simulink model "six_plus_six_AcmsteeringV09_main_2lfrf"  (R2014a)
settings: Solver=FixedStepDiscrete  StartTime=0.0  StopTime=10.0  FixedStep=0.0005  RelTol=1e-3
InitFcn:
  | Veh_Par_wxt
undefined symbols (not defined in the file or in its folder): acc_spdctl, ag_thr, B, bra_em, bra_pre_gz2, bra_pre_gz34, bra_pre_yd, brakepre_dem_data, brakeTrq_dem_data, bratrq_max, ecucoder_acal, eff_tran, ESP_switch, G, guzhang_lf, guzhang_lm, guzhang_lr, guzhang_rf, guzhang_rm, guzhang_rr, kd1, kd2, ki1, ki2, kp1, kp2, L, myFIS, premax, Radius, RC_switch, s_opt_yi, s_opt_zhuan, s_opt_zhuan_add, s_opt_zhuan_table, spd_map_mot, spd_spdctl, speed_thr_park, TCS_switch, tras_ratio, trq_map_mot, trqmax_yd, trqmax_zx, trqmaxneg, v_gain, v_table, v_thr_park, zhidong_bianmazhi, zhidong_down, zhidong_up, zhidong_youmen, zhuanxiang_bianmazhi, zhuanxiang_down, zhuanxiang_up, zhuanxiang_youmen
libraries: simulink x980, ec5744lib x59, fuzblock x2
(part 14 of 25)

== matlab function six_plus_six_AcmsteeringV09_main_2lfrf/Subsystem/MATLAB Function3 ==
  data: data_1 input; data output; data_2 input; zero output; position_4 output; position_3 output; position_2 output; position_1 output
function [data,zero,position_4,position_3,position_2,position_1] = motec_write(data_1,data_2)
if  data_1<150
    if (mod(data_1,6)<3)
    data=6;
    else
    data=7;
    end
    zero=hex2dec('00');
    position_1=hex2dec('00');
    position_2=hex2dec('00');
    position_3=hex2dec('00');
    position_4=hex2dec('00');  
else
    if (mod(data_1,2)==0)
        data=15;
        zero=hex2dec('00');
    else
        zero=hex2dec('00');
        data=95;    
    end
%Negative numbers are represented with the Two's Complement
       data_2=double(data_2);
       if data_2<0
       data_2= 2^32+data_2;
       end
%Find the 4 bytes
       position_1= floor( data_2/(2^24) );
       remainder1     = floor( mod( data_2,(2^24) ) );
       position_2= floor( remainder1/(2^16) );
       remainder2     = floor( mod( remainder1,(2^16) ) );
       position_3= floor( remainder2/(2^8) );
       position_4= floor( mod( remainder2,(2^8) ) );
 
end

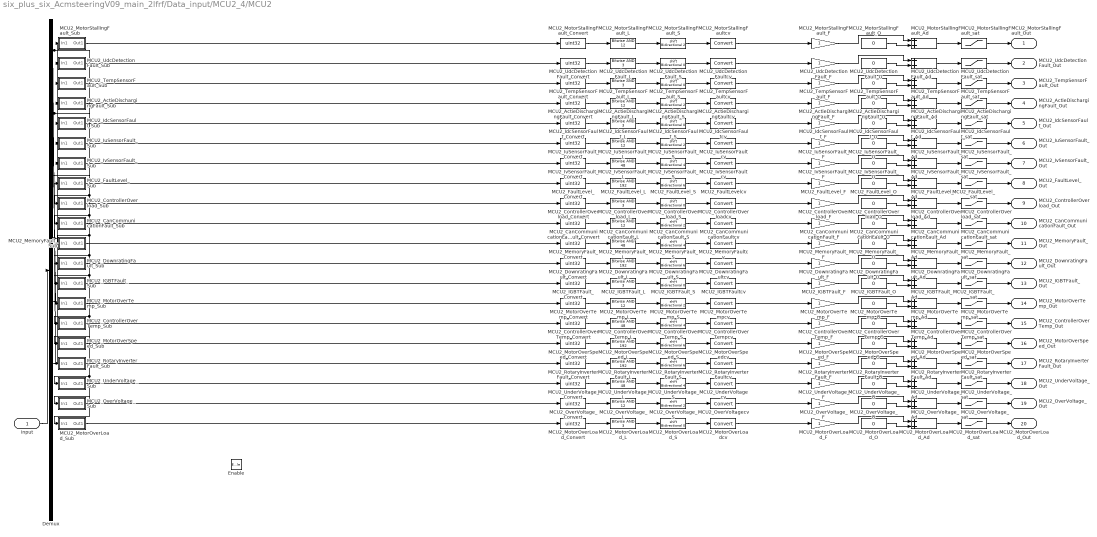
== system six_plus_six_AcmsteeringV09_main_2lfrf/Data_input/MCU2_4/MCU2 ==
  input : Inport
  Enable : EnablePort
  Demux : Demux  Outputs=8
  MCU2_ActieDischargingFault_Ad : Sum
  MCU2_ActieDischargingFault_Convert : DataTypeConversion  OutDataTypeStr=uint32
  MCU2_ActieDischargingFault_F : Gain
  MCU2_ActieDischargingFault_L : simulink/Logic and Bit Operations/Bitwise Operator  logicop=AND  UseBitMask=on  BitMask=12  BitMaskRealWorld=Stored Integer
  MCU2_ActieDischargingFault_O : Constant  Value=0  OutDataTypeStr=single
  MCU2_ActieDischargingFault_S : ArithShift  BitShiftNumber=2
  MCU2_ActieDischargingFault_Sub : Subsystem
  MCU2_ActieDischargingFault_sat : Saturate  UpperLimit=3  LowerLimit=0
  MCU2_ActieDischargingFaultcv : DataTypeConversion
  MCU2_CanCommunicationFault_Ad : Sum
  MCU2_CanCommunicationFault_Convert : DataTypeConversion  OutDataTypeStr=uint32
  MCU2_CanCommunicationFault_F : Gain
  MCU2_CanCommunicationFault_L : simulink/Logic and Bit Operations/Bitwise Operator  logicop=AND  UseBitMask=on  BitMask=12  BitMaskRealWorld=Stored Integer
  MCU2_CanCommunicationFault_O : Constant  Value=0  OutDataTypeStr=single
  MCU2_CanCommunicationFault_S : ArithShift  BitShiftNumber=2
  MCU2_CanCommunicationFault_Sub : Subsystem
  MCU2_CanCommunicationFault_sat : Saturate  UpperLimit=3  LowerLimit=0
  MCU2_CanCommunicationFaultcv : DataTypeConversion
  MCU2_ControllerOverTemp_Ad : Sum
  MCU2_ControllerOverTemp_Convert : DataTypeConversion  OutDataTypeStr=uint32
  MCU2_ControllerOverTemp_F : Gain
  MCU2_ControllerOverTemp_L : simulink/Logic and Bit Operations/Bitwise Operator  logicop=AND  UseBitMask=on  BitMask=48  BitMaskRealWorld=Stored Integer
  MCU2_ControllerOverTemp_O : Constant  Value=0  OutDataTypeStr=single
  MCU2_ControllerOverTemp_S : ArithShift  BitShiftNumber=4
  MCU2_ControllerOverTemp_Sub : Subsystem
  MCU2_ControllerOverTemp_sat : Saturate  UpperLimit=3  LowerLimit=0
  MCU2_ControllerOverTempcv : DataTypeConversion
  MCU2_ControllerOverload_Ad : Sum
  MCU2_ControllerOverload_Convert : DataTypeConversion  OutDataTypeStr=uint32
  MCU2_ControllerOverload_F : Gain
  MCU2_ControllerOverload_L : simulink/Logic and Bit Operations/Bitwise Operator  logicop=AND  UseBitMask=on  BitMask=3  BitMaskRealWorld=Stored Integer
  MCU2_ControllerOverload_O : Constant  Value=0  OutDataTypeStr=single
  MCU2_ControllerOverload_S : ArithShift
  MCU2_ControllerOverload_Sub : Subsystem
  MCU2_ControllerOverload_sat : Saturate  UpperLimit=3  LowerLimit=0
  MCU2_ControllerOverloadcv : DataTypeConversion
  MCU2_DownratingFault_Ad : Sum
  MCU2_DownratingFault_Convert : DataTypeConversion  OutDataTypeStr=uint32
  MCU2_DownratingFault_F : Gain
  MCU2_DownratingFault_L : simulink/Logic and Bit Operations/Bitwise Operator  logicop=AND  UseBitMask=on  BitMask=192  BitMaskRealWorld=Stored Integer
  MCU2_DownratingFault_O : Constant  Value=0  OutDataTypeStr=single
  MCU2_DownratingFault_S : ArithShift  BitShiftNumber=6
  MCU2_DownratingFault_Sub : Subsystem
  MCU2_DownratingFault_sat : Saturate  UpperLimit=3  LowerLimit=0
  MCU2_DownratingFaultcv : DataTypeConversion
  MCU2_FaultLevel_Ad : Sum
  MCU2_FaultLevel_Convert : DataTypeConversion  OutDataTypeStr=uint32
  MCU2_FaultLevel_F : Gain
  MCU2_FaultLevel_L : simulink/Logic and Bit Operations/Bitwise Operator  logicop=AND  UseBitMask=on  BitMask=192  BitMaskRealWorld=Stored Integer
  MCU2_FaultLevel_O : Constant  Value=0  OutDataTypeStr=single
  MCU2_FaultLevel_S : ArithShift  BitShiftNumber=6
  MCU2_FaultLevel_Sub : Subsystem
  MCU2_FaultLevel_sat : Saturate  UpperLimit=3  LowerLimit=0
  MCU2_FaultLevelcv : DataTypeConversion
  MCU2_IGBTFault_Ad : Sum
  MCU2_IGBTFault_Convert : DataTypeConversion  OutDataTypeStr=uint32
  MCU2_IGBTFault_F : Gain
  MCU2_IGBTFault_L : simulink/Logic and Bit Operations/Bitwise Operator  logicop=AND  UseBitMask=on  BitMask=3  BitMaskRealWorld=Stored Integer
  MCU2_IGBTFault_O : Constant  Value=0  OutDataTypeStr=single
  MCU2_IGBTFault_S : ArithShift
  MCU2_IGBTFault_Sub : Subsystem
  MCU2_IGBTFault_sat : Saturate  UpperLimit=3  LowerLimit=0
  MCU2_IGBTFaultcv : DataTypeConversion
  MCU2_IdcSensorFault_Ad : Sum
  MCU2_IdcSensorFault_Convert : DataTypeConversion  OutDataTypeStr=uint32
  MCU2_IdcSensorFault_F : Gain
  MCU2_IdcSensorFault_L : simulink/Logic and Bit Operations/Bitwise Operator  logicop=AND  UseBitMask=on  BitMask=3  BitMaskRealWorld=Stored Integer
  MCU2_IdcSensorFault_O : Constant  Value=0  OutDataTypeStr=single
  MCU2_IdcSensorFault_S : ArithShift
  MCU2_IdcSensorFault_Sub : Subsystem
  MCU2_IdcSensorFault_sat : Saturate  UpperLimit=3  LowerLimit=0
  MCU2_IdcSensorFaultcv : DataTypeConversion
  MCU2_IuSensorFault_Ad : Sum
  MCU2_IuSensorFault_Convert : DataTypeConversion  OutDataTypeStr=uint32
  MCU2_IuSensorFault_F : Gain
  MCU2_IuSensorFault_L : simulink/Logic and Bit Operations/Bitwise Operator  logicop=AND  UseBitMask=on  BitMask=12  BitMaskRealWorld=Stored Integer
  MCU2_IuSensorFault_O : Constant  Value=0  OutDataTypeStr=single
  MCU2_IuSensorFault_S : ArithShift  BitShiftNumber=2
  MCU2_IuSensorFault_Sub : Subsystem
  MCU2_IuSensorFault_sat : Saturate  UpperLimit=3  LowerLimit=0
  MCU2_IuSensorFaultcv : DataTypeConversion
  MCU2_IvSensorFault_Ad : Sum
  MCU2_IvSensorFault_Convert : DataTypeConversion  OutDataTypeStr=uint32
  MCU2_IvSensorFault_F : Gain
  MCU2_IvSensorFault_L : simulink/Logic and Bit Operations/Bitwise Operator  logicop=AND  UseBitMask=on  BitMask=48  BitMaskRealWorld=Stored Integer
  MCU2_IvSensorFault_O : Constant  Value=0  OutDataTypeStr=single
  MCU2_IvSensorFault_S : ArithShift  BitShiftNumber=4
  MCU2_IvSensorFault_Sub : Subsystem
  MCU2_IvSensorFault_sat : Saturate  UpperLimit=3  LowerLimit=0
  MCU2_IvSensorFaultcv : DataTypeConversion
  MCU2_MemoryFault_Ad : Sum
  MCU2_MemoryFault_Convert : DataTypeConversion  OutDataTypeStr=uint32
  MCU2_MemoryFault_F : Gain
  MCU2_MemoryFault_L : simulink/Logic and Bit Operations/Bitwise Operator  logicop=AND  UseBitMask=on  BitMask=48  BitMaskRealWorld=Stored Integer
  MCU2_MemoryFault_O : Constant  Value=0  OutDataTypeStr=single
  MCU2_MemoryFault_S : ArithShift  BitShiftNumber=4
  MCU2_MemoryFault_Sub : Subsystem
  MCU2_MemoryFault_sat : Saturate  UpperLimit=3  LowerLimit=0
  MCU2_MemoryFaultcv : DataTypeConversion
  MCU2_MotorOverLoad_Ad : Sum
  MCU2_MotorOverLoad_Convert : DataTypeConversion  OutDataTypeStr=uint32
  MCU2_MotorOverLoad_F : Gain
  MCU2_MotorOverLoad_L : simulink/Logic and Bit Operations/Bitwise Operator  logicop=AND  UseBitMask=on  BitMask=3  BitMaskRealWorld=Stored Integer
  MCU2_MotorOverLoad_O : Constant  Value=0  OutDataTypeStr=single
  MCU2_MotorOverLoad_S : ArithShift
  MCU2_MotorOverLoad_Sub : Subsystem
  MCU2_MotorOverLoad_sat : Saturate  UpperLimit=3  LowerLimit=0
  MCU2_MotorOverLoadcv : DataTypeConversion
  MCU2_MotorOverSpeed_Ad : Sum
  MCU2_MotorOverSpeed_Convert : DataTypeConversion  OutDataTypeStr=uint32
  MCU2_MotorOverSpeed_F : Gain
  MCU2_MotorOverSpeed_L : simulink/Logic and Bit Operations/Bitwise Operator  logicop=AND  UseBitMask=on  BitMask=192  BitMaskRealWorld=Stored Integer
  MCU2_MotorOverSpeed_O : Constant  Value=0  OutDataTypeStr=single
  MCU2_MotorOverSpeed_S : ArithShift  BitShiftNumber=6
  MCU2_MotorOverSpeed_Sub : Subsystem
  MCU2_MotorOverSpeed_sat : Saturate  UpperLimit=3  LowerLimit=0
  MCU2_MotorOverSpeedcv : DataTypeConversion
  MCU2_MotorOverTemp_Ad : Sum
  MCU2_MotorOverTemp_Convert : DataTypeConversion  OutDataTypeStr=uint32
  MCU2_MotorOverTemp_F : Gain
  MCU2_MotorOverTemp_L : simulink/Logic and Bit Operations/Bitwise Operator  logicop=AND  UseBitMask=on  BitMask=12  BitMaskRealWorld=Stored Integer
  MCU2_MotorOverTemp_O : Constant  Value=0  OutDataTypeStr=single
  MCU2_MotorOverTemp_S : ArithShift  BitShiftNumber=2
  MCU2_MotorOverTemp_Sub : Subsystem
  MCU2_MotorOverTemp_sat : Saturate  UpperLimit=3  LowerLimit=0
  MCU2_MotorOverTempcv : DataTypeConversion
  MCU2_MotorStallingFault_Ad : Sum
  MCU2_MotorStallingFault_Convert : DataTypeConversion  OutDataTypeStr=uint32
  MCU2_MotorStallingFault_F : Gain
  MCU2_MotorStallingFault_L : simulink/Logic and Bit Operations/Bitwise Operator  logicop=AND  UseBitMask=on  BitMask=12  BitMaskRealWorld=Stored Integer
  MCU2_MotorStallingFault_O : Constant  Value=0  OutDataTypeStr=single
  MCU2_MotorStallingFault_S : ArithShift  BitShiftNumber=2
  MCU2_MotorStallingFault_Sub : Subsystem
  MCU2_MotorStallingFault_sat : Saturate  UpperLimit=3  LowerLimit=0
  MCU2_MotorStallingFaultcv : DataTypeConversion
  MCU2_OverVoltage_Ad : Sum
  MCU2_OverVoltage_Convert : DataTypeConversion  OutDataTypeStr=uint32
  MCU2_OverVoltage_F : Gain
  MCU2_OverVoltage_L : simulink/Logic and Bit Operations/Bitwise Operator  logicop=AND  UseBitMask=on  BitMask=12  BitMaskRealWorld=Stored Integer
  MCU2_OverVoltage_O : Constant  Value=0  OutDataTypeStr=single
  MCU2_OverVoltage_S : ArithShift  BitShiftNumber=2
  MCU2_OverVoltage_Sub : Subsystem
  MCU2_OverVoltage_sat : Saturate  UpperLimit=3  LowerLimit=0
  MCU2_OverVoltagecv : DataTypeConversion
  MCU2_RotaryInverterFault_Ad : Sum
  MCU2_RotaryInverterFault_Convert : DataTypeConversion  OutDataTypeStr=uint32
  MCU2_RotaryInverterFault_F : Gain
  MCU2_RotaryInverterFault_L : simulink/Logic and Bit Operations/Bitwise Operator  logicop=AND  UseBitMask=on  BitMask=192  BitMaskRealWorld=Stored Integer
  MCU2_RotaryInverterFault_O : Constant  Value=0  OutDataTypeStr=single
  MCU2_RotaryInverterFault_S : ArithShift  BitShiftNumber=6
  MCU2_RotaryInverterFault_Sub : Subsystem
  MCU2_RotaryInverterFault_sat : Saturate  UpperLimit=3  LowerLimit=0
  MCU2_RotaryInverterFaultcv : DataTypeConversion
  MCU2_TempSensorFault_Ad : Sum
  MCU2_TempSensorFault_Convert : DataTypeConversion  OutDataTypeStr=uint32
  MCU2_TempSensorFault_F : Gain
  MCU2_TempSensorFault_L : simulink/Logic and Bit Operations/Bitwise Operator  logicop=AND  UseBitMask=on  BitMask=3  BitMaskRealWorld=Stored Integer
  MCU2_TempSensorFault_O : Constant  Value=0  OutDataTypeStr=single
  MCU2_TempSensorFault_S : ArithShift
  MCU2_TempSensorFault_Sub : Subsystem
  MCU2_TempSensorFault_sat : Saturate  UpperLimit=3  LowerLimit=0
  MCU2_TempSensorFaultcv : DataTypeConversion
  MCU2_UdcDetectionFault_Ad : Sum
  MCU2_UdcDetectionFault_Convert : DataTypeConversion  OutDataTypeStr=uint32
  MCU2_UdcDetectionFault_F : Gain
  MCU2_UdcDetectionFault_L : simulink/Logic and Bit Operations/Bitwise Operator  logicop=AND  UseBitMask=on  BitMask=3  BitMaskRealWorld=Stored Integer
  MCU2_UdcDetectionFault_O : Constant  Value=0  OutDataTypeStr=single
  MCU2_UdcDetectionFault_S : ArithShift
  MCU2_UdcDetectionFault_Sub : Subsystem
  MCU2_UdcDetectionFault_sat : Saturate  UpperLimit=3  LowerLimit=0
  MCU2_UdcDetectionFaultcv : DataTypeConversion
  MCU2_UnderVoltage_Ad : Sum
  MCU2_UnderVoltage_Convert : DataTypeConversion  OutDataTypeStr=uint32
  MCU2_UnderVoltage_F : Gain
  MCU2_UnderVoltage_L : simulink/Logic and Bit Operations/Bitwise Operator  logicop=AND  UseBitMask=on  BitMask=48  BitMaskRealWorld=Stored Integer
  MCU2_UnderVoltage_O : Constant  Value=0  OutDataTypeStr=single
  MCU2_UnderVoltage_S : ArithShift  BitShiftNumber=4
  MCU2_UnderVoltage_Sub : Subsystem
  MCU2_UnderVoltage_sat : Saturate  UpperLimit=3  LowerLimit=0
  MCU2_UnderVoltagecv : DataTypeConversion
  MCU2_MotorStallingFault_Out : Outport
  MCU2_UdcDetectionFault_Out : Outport  Port=2
  MCU2_TempSensorFault_Out : Outport  Port=3
  MCU2_ActieDischargingFault_Out : Outport  Port=4
  MCU2_IdcSensorFault_Out : Outport  Port=5
  MCU2_IuSensorFault_Out : Outport  Port=6
  MCU2_IvSensorFault_Out : Outport  Port=7
  MCU2_FaultLevel_Out : Outport  Port=8
  MCU2_ControllerOverload_Out : Outport  Port=9
  MCU2_CanCommunicationFault_Out : Outport  Port=10
  MCU2_MemoryFault_Out : Outport  Port=11
  MCU2_DownratingFault_Out : Outport  Port=12
  MCU2_IGBTFault_Out : Outport  Port=13
  MCU2_MotorOverTemp_Out : Outport  Port=14
  MCU2_ControllerOverTemp_Out : Outport  Port=15
  MCU2_MotorOverSpeed_Out : Outport  Port=16
  MCU2_RotaryInverterFault_Out : Outport  Port=17
  MCU2_UnderVoltage_Out : Outport  Port=18
  MCU2_OverVoltage_Out : Outport  Port=19
  MCU2_MotorOverLoad_Out : Outport  Port=20
  wires:
  MCU2_MotorStallingFault_F/1 -> MCU2_MotorStallingFault_Ad/1
  MCU2_MotorStallingFault_O/1 -> MCU2_MotorStallingFault_Ad/2
  MCU2_MotorStallingFault_Ad/1 -> MCU2_MotorStallingFault_sat/1
  MCU2_MotorStallingFault_sat/1 -> MCU2_MotorStallingFault_Out/1
  Demux/6 -> MCU2_MotorStallingFault_Sub/1(In1), MCU2_UdcDetectionFault_Sub/1(In1)
  MCU2_MotorStallingFault_Sub/1(Out1) -> MCU2_MotorStallingFault_Convert/1
  MCU2_MotorStallingFault_Convert/1 -> MCU2_MotorStallingFault_L/1
  MCU2_MotorStallingFault_L/1 -> MCU2_MotorStallingFault_S/1
  MCU2_MotorStallingFault_S/1 -> MCU2_MotorStallingFaultcv/1
  MCU2_MotorStallingFaultcv/1 -> MCU2_MotorStallingFault_F/1
  MCU2_UdcDetectionFault_F/1 -> MCU2_UdcDetectionFault_Ad/1
  MCU2_UdcDetectionFault_O/1 -> MCU2_UdcDetectionFault_Ad/2
  MCU2_UdcDetectionFault_Ad/1 -> MCU2_UdcDetectionFault_sat/1
  MCU2_UdcDetectionFault_sat/1 -> MCU2_UdcDetectionFault_Out/1
  MCU2_UdcDetectionFault_Sub/1(Out1) -> MCU2_UdcDetectionFault_Convert/1
  MCU2_UdcDetectionFault_Convert/1 -> MCU2_UdcDetectionFault_L/1
  MCU2_UdcDetectionFault_L/1 -> MCU2_UdcDetectionFault_S/1
  MCU2_UdcDetectionFault_S/1 -> MCU2_UdcDetectionFaultcv/1
  MCU2_UdcDetectionFaultcv/1 -> MCU2_UdcDetectionFault_F/1
  MCU2_TempSensorFault_F/1 -> MCU2_TempSensorFault_Ad/1
  MCU2_TempSensorFault_O/1 -> MCU2_TempSensorFault_Ad/2
  MCU2_TempSensorFault_Ad/1 -> MCU2_TempSensorFault_sat/1
  MCU2_TempSensorFault_sat/1 -> MCU2_TempSensorFault_Out/1
  Demux/5 -> MCU2_TempSensorFault_Sub/1(In1), MCU2_ActieDischargingFault_Sub/1(In1)
  MCU2_TempSensorFault_Sub/1(Out1) -> MCU2_TempSensorFault_Convert/1
  MCU2_TempSensorFault_Convert/1 -> MCU2_TempSensorFault_L/1
  MCU2_TempSensorFault_L/1 -> MCU2_TempSensorFault_S/1
  MCU2_TempSensorFault_S/1 -> MCU2_TempSensorFaultcv/1
  MCU2_TempSensorFaultcv/1 -> MCU2_TempSensorFault_F/1
  MCU2_ActieDischargingFault_F/1 -> MCU2_ActieDischargingFault_Ad/1
  MCU2_ActieDischargingFault_O/1 -> MCU2_ActieDischargingFault_Ad/2
  MCU2_ActieDischargingFault_Ad/1 -> MCU2_ActieDischargingFault_sat/1
  MCU2_ActieDischargingFault_sat/1 -> MCU2_ActieDischargingFault_Out/1
  MCU2_ActieDischargingFault_Sub/1(Out1) -> MCU2_ActieDischargingFault_Convert/1
  MCU2_ActieDischargingFault_Convert/1 -> MCU2_ActieDischargingFault_L/1
  MCU2_ActieDischargingFault_L/1 -> MCU2_ActieDischargingFault_S/1
  MCU2_ActieDischargingFault_S/1 -> MCU2_ActieDischargingFaultcv/1
  MCU2_ActieDischargingFaultcv/1 -> MCU2_ActieDischargingFault_F/1
  MCU2_IdcSensorFault_F/1 -> MCU2_IdcSensorFault_Ad/1
  MCU2_IdcSensorFault_O/1 -> MCU2_IdcSensorFault_Ad/2
  MCU2_IdcSensorFault_Ad/1 -> MCU2_IdcSensorFault_sat/1
  MCU2_IdcSensorFault_sat/1 -> MCU2_IdcSensorFault_Out/1
  Demux/4 -> MCU2_IdcSensorFault_Sub/1(In1), MCU2_IuSensorFault_Sub/1(In1), MCU2_IvSensorFault_Sub/1(In1), MCU2_FaultLevel_Sub/1(In1)
  MCU2_IdcSensorFault_Sub/1(Out1) -> MCU2_IdcSensorFault_Convert/1
  MCU2_IdcSensorFault_Convert/1 -> MCU2_IdcSensorFault_L/1
  MCU2_IdcSensorFault_L/1 -> MCU2_IdcSensorFault_S/1
  MCU2_IdcSensorFault_S/1 -> MCU2_IdcSensorFaultcv/1
  MCU2_IdcSensorFaultcv/1 -> MCU2_IdcSensorFault_F/1
  MCU2_IuSensorFault_F/1 -> MCU2_IuSensorFault_Ad/1
  MCU2_IuSensorFault_O/1 -> MCU2_IuSensorFault_Ad/2
  MCU2_IuSensorFault_Ad/1 -> MCU2_IuSensorFault_sat/1
  MCU2_IuSensorFault_sat/1 -> MCU2_IuSensorFault_Out/1
  MCU2_IuSensorFault_Sub/1(Out1) -> MCU2_IuSensorFault_Convert/1
  MCU2_IuSensorFault_Convert/1 -> MCU2_IuSensorFault_L/1
  MCU2_IuSensorFault_L/1 -> MCU2_IuSensorFault_S/1
  MCU2_IuSensorFault_S/1 -> MCU2_IuSensorFaultcv/1
  MCU2_IuSensorFaultcv/1 -> MCU2_IuSensorFault_F/1
  MCU2_IvSensorFault_F/1 -> MCU2_IvSensorFault_Ad/1
  MCU2_IvSensorFault_O/1 -> MCU2_IvSensorFault_Ad/2
  MCU2_IvSensorFault_Ad/1 -> MCU2_IvSensorFault_sat/1
  MCU2_IvSensorFault_sat/1 -> MCU2_IvSensorFault_Out/1
  MCU2_IvSensorFault_Sub/1(Out1) -> MCU2_IvSensorFault_Convert/1
  MCU2_IvSensorFault_Convert/1 -> MCU2_IvSensorFault_L/1
  MCU2_IvSensorFault_L/1 -> MCU2_IvSensorFault_S/1
  MCU2_IvSensorFault_S/1 -> MCU2_IvSensorFaultcv/1
  MCU2_IvSensorFaultcv/1 -> MCU2_IvSensorFault_F/1
  MCU2_FaultLevel_F/1 -> MCU2_FaultLevel_Ad/1
  MCU2_FaultLevel_O/1 -> MCU2_FaultLevel_Ad/2
  MCU2_FaultLevel_Ad/1 -> MCU2_FaultLevel_sat/1
  MCU2_FaultLevel_sat/1 -> MCU2_FaultLevel_Out/1
  MCU2_FaultLevel_Sub/1(Out1) -> MCU2_FaultLevel_Convert/1
  MCU2_FaultLevel_Convert/1 -> MCU2_FaultLevel_L/1
  MCU2_FaultLevel_L/1 -> MCU2_FaultLevel_S/1
  MCU2_FaultLevel_S/1 -> MCU2_FaultLevelcv/1
  MCU2_FaultLevelcv/1 -> MCU2_FaultLevel_F/1
  MCU2_ControllerOverload_F/1 -> MCU2_ControllerOverload_Ad/1
  MCU2_ControllerOverload_O/1 -> MCU2_ControllerOverload_Ad/2
  MCU2_ControllerOverload_Ad/1 -> MCU2_ControllerOverload_sat/1
  MCU2_ControllerOverload_sat/1 -> MCU2_ControllerOverload_Out/1
  Demux/1 -> MCU2_UnderVoltage_Sub/1(In1), MCU2_OverVoltage_Sub/1(In1), MCU2_ControllerOverload_Sub/1(In1), MCU2_RotaryInverterFault_Sub/1(In1)
  MCU2_ControllerOverload_Sub/1(Out1) -> MCU2_ControllerOverload_Convert/1
  MCU2_ControllerOverload_Convert/1 -> MCU2_ControllerOverload_L/1
  MCU2_ControllerOverload_L/1 -> MCU2_ControllerOverload_S/1
  MCU2_ControllerOverload_S/1 -> MCU2_ControllerOverloadcv/1
  MCU2_ControllerOverloadcv/1 -> MCU2_ControllerOverload_F/1
  MCU2_CanCommunicationFault_F/1 -> MCU2_CanCommunicationFault_Ad/1
  MCU2_CanCommunicationFault_O/1 -> MCU2_CanCommunicationFault_Ad/2
  MCU2_CanCommunicationFault_Ad/1 -> MCU2_CanCommunicationFault_sat/1
  MCU2_CanCommunicationFault_sat/1 -> MCU2_CanCommunicationFault_Out/1
  Demux/3 -> MCU2_DownratingFault_Sub/1(In1), MCU2_MotorOverLoad_Sub/1(In1), MCU2_MemoryFault_Sub/1(In1), MCU2_CanCommunicationFault_Sub/1(In1)
  MCU2_CanCommunicationFault_Sub/1(Out1) -> MCU2_CanCommunicationFault_Convert/1
  MCU2_CanCommunicationFault_Convert/1 -> MCU2_CanCommunicationFault_L/1
  MCU2_CanCommunicationFault_L/1 -> MCU2_CanCommunicationFault_S/1
  MCU2_CanCommunicationFault_S/1 -> MCU2_CanCommunicationFaultcv/1
  MCU2_CanCommunicationFaultcv/1 -> MCU2_CanCommunicationFault_F/1
  MCU2_MemoryFault_F/1 -> MCU2_MemoryFault_Ad/1
  MCU2_MemoryFault_O/1 -> MCU2_MemoryFault_Ad/2
  MCU2_MemoryFault_Ad/1 -> MCU2_MemoryFault_sat/1
  MCU2_MemoryFault_sat/1 -> MCU2_MemoryFault_Out/1
  MCU2_MemoryFault_Sub/1(Out1) -> MCU2_MemoryFault_Convert/1
  MCU2_MemoryFault_Convert/1 -> MCU2_MemoryFault_L/1
  MCU2_MemoryFault_L/1 -> MCU2_MemoryFault_S/1
  MCU2_MemoryFault_S/1 -> MCU2_MemoryFaultcv/1
  MCU2_MemoryFaultcv/1 -> MCU2_MemoryFault_F/1
  MCU2_DownratingFault_F/1 -> MCU2_DownratingFault_Ad/1
  MCU2_DownratingFault_O/1 -> MCU2_DownratingFault_Ad/2
  MCU2_DownratingFault_Ad/1 -> MCU2_DownratingFault_sat/1
  MCU2_DownratingFault_sat/1 -> MCU2_DownratingFault_Out/1
  MCU2_DownratingFault_Sub/1(Out1) -> MCU2_DownratingFault_Convert/1
  MCU2_DownratingFault_Convert/1 -> MCU2_DownratingFault_L/1
  MCU2_DownratingFault_L/1 -> MCU2_DownratingFault_S/1
  MCU2_DownratingFault_S/1 -> MCU2_DownratingFaultcv/1
  MCU2_DownratingFaultcv/1 -> MCU2_DownratingFault_F/1
  MCU2_IGBTFault_F/1 -> MCU2_IGBTFault_Ad/1
  MCU2_IGBTFault_O/1 -> MCU2_IGBTFault_Ad/2
  MCU2_IGBTFault_Ad/1 -> MCU2_IGBTFault_sat/1
  MCU2_IGBTFault_sat/1 -> MCU2_IGBTFault_Out/1
  Demux/2 -> MCU2_ControllerOverTemp_Sub/1(In1), MCU2_MotorOverSpeed_Sub/1(In1), MCU2_IGBTFault_Sub/1(In1), MCU2_MotorOverTemp_Sub/1(In1)
  MCU2_IGBTFault_Sub/1(Out1) -> MCU2_IGBTFault_Convert/1
  MCU2_IGBTFault_Convert/1 -> MCU2_IGBTFault_L/1
  MCU2_IGBTFault_L/1 -> MCU2_IGBTFault_S/1
  MCU2_IGBTFault_S/1 -> MCU2_IGBTFaultcv/1
  MCU2_IGBTFaultcv/1 -> MCU2_IGBTFault_F/1
  MCU2_MotorOverTemp_F/1 -> MCU2_MotorOverTemp_Ad/1
  MCU2_MotorOverTemp_O/1 -> MCU2_MotorOverTemp_Ad/2
  MCU2_MotorOverTemp_Ad/1 -> MCU2_MotorOverTemp_sat/1
  MCU2_MotorOverTemp_sat/1 -> MCU2_MotorOverTemp_Out/1
  MCU2_MotorOverTemp_Sub/1(Out1) -> MCU2_MotorOverTemp_Convert/1
  MCU2_MotorOverTemp_Convert/1 -> MCU2_MotorOverTemp_L/1
  MCU2_MotorOverTemp_L/1 -> MCU2_MotorOverTemp_S/1
  MCU2_MotorOverTemp_S/1 -> MCU2_MotorOverTempcv/1
  MCU2_MotorOverTempcv/1 -> MCU2_MotorOverTemp_F/1
  MCU2_ControllerOverTemp_F/1 -> MCU2_ControllerOverTemp_Ad/1
  MCU2_ControllerOverTemp_O/1 -> MCU2_ControllerOverTemp_Ad/2
  MCU2_ControllerOverTemp_Ad/1 -> MCU2_ControllerOverTemp_sat/1
  MCU2_ControllerOverTemp_sat/1 -> MCU2_ControllerOverTemp_Out/1
  MCU2_ControllerOverTemp_Sub/1(Out1) -> MCU2_ControllerOverTemp_Convert/1
  MCU2_ControllerOverTemp_Convert/1 -> MCU2_ControllerOverTemp_L/1
  MCU2_ControllerOverTemp_L/1 -> MCU2_ControllerOverTemp_S/1
  MCU2_ControllerOverTemp_S/1 -> MCU2_ControllerOverTempcv/1
  MCU2_ControllerOverTempcv/1 -> MCU2_ControllerOverTemp_F/1
  MCU2_MotorOverSpeed_F/1 -> MCU2_MotorOverSpeed_Ad/1
  MCU2_MotorOverSpeed_O/1 -> MCU2_MotorOverSpeed_Ad/2
  MCU2_MotorOverSpeed_Ad/1 -> MCU2_MotorOverSpeed_sat/1
  MCU2_MotorOverSpeed_sat/1 -> MCU2_MotorOverSpeed_Out/1
  MCU2_MotorOverSpeed_Sub/1(Out1) -> MCU2_MotorOverSpeed_Convert/1
  MCU2_MotorOverSpeed_Convert/1 -> MCU2_MotorOverSpeed_L/1
  MCU2_MotorOverSpeed_L/1 -> MCU2_MotorOverSpeed_S/1
  MCU2_MotorOverSpeed_S/1 -> MCU2_MotorOverSpeedcv/1
  MCU2_MotorOverSpeedcv/1 -> MCU2_MotorOverSpeed_F/1
  MCU2_RotaryInverterFault_F/1 -> MCU2_RotaryInverterFault_Ad/1
  MCU2_RotaryInverterFault_O/1 -> MCU2_RotaryInverterFault_Ad/2
  MCU2_RotaryInverterFault_Ad/1 -> MCU2_RotaryInverterFault_sat/1
  MCU2_RotaryInverterFault_sat/1 -> MCU2_RotaryInverterFault_Out/1
  MCU2_RotaryInverterFault_Sub/1(Out1) -> MCU2_RotaryInverterFault_Convert/1
  MCU2_RotaryInverterFault_Convert/1 -> MCU2_RotaryInverterFault_L/1
  MCU2_RotaryInverterFault_L/1 -> MCU2_RotaryInverterFault_S/1
  MCU2_RotaryInverterFault_S/1 -> MCU2_RotaryInverterFaultcv/1
  MCU2_RotaryInverterFaultcv/1 -> MCU2_RotaryInverterFault_F/1
  MCU2_UnderVoltage_F/1 -> MCU2_UnderVoltage_Ad/1
  MCU2_UnderVoltage_O/1 -> MCU2_UnderVoltage_Ad/2
  MCU2_UnderVoltage_Ad/1 -> MCU2_UnderVoltage_sat/1
  MCU2_UnderVoltage_sat/1 -> MCU2_UnderVoltage_Out/1
  MCU2_UnderVoltage_Sub/1(Out1) -> MCU2_UnderVoltage_Convert/1
  MCU2_UnderVoltage_Convert/1 -> MCU2_UnderVoltage_L/1
  MCU2_UnderVoltage_L/1 -> MCU2_UnderVoltage_S/1
  MCU2_UnderVoltage_S/1 -> MCU2_UnderVoltagecv/1
  MCU2_UnderVoltagecv/1 -> MCU2_UnderVoltage_F/1
  MCU2_OverVoltage_F/1 -> MCU2_OverVoltage_Ad/1
  MCU2_OverVoltage_O/1 -> MCU2_OverVoltage_Ad/2
  MCU2_OverVoltage_Ad/1 -> MCU2_OverVoltage_sat/1
  MCU2_OverVoltage_sat/1 -> MCU2_OverVoltage_Out/1
  MCU2_OverVoltage_Sub/1(Out1) -> MCU2_OverVoltage_Convert/1
  MCU2_OverVoltage_Convert/1 -> MCU2_OverVoltage_L/1
  MCU2_OverVoltage_L/1 -> MCU2_OverVoltage_S/1
  MCU2_OverVoltage_S/1 -> MCU2_OverVoltagecv/1
  MCU2_OverVoltagecv/1 -> MCU2_OverVoltage_F/1
  MCU2_MotorOverLoad_F/1 -> MCU2_MotorOverLoad_Ad/1
  MCU2_MotorOverLoad_O/1 -> MCU2_MotorOverLoad_Ad/2
  MCU2_MotorOverLoad_Ad/1 -> MCU2_MotorOverLoad_sat/1
  MCU2_MotorOverLoad_sat/1 -> MCU2_MotorOverLoad_Out/1
  MCU2_MotorOverLoad_Sub/1(Out1) -> MCU2_MotorOverLoad_Convert/1
  MCU2_MotorOverLoad_Convert/1 -> MCU2_MotorOverLoad_L/1
  MCU2_MotorOverLoad_L/1 -> MCU2_MotorOverLoad_S/1
  MCU2_MotorOverLoad_S/1 -> MCU2_MotorOverLoadcv/1
  MCU2_MotorOverLoadcv/1 -> MCU2_MotorOverLoad_F/1
  input/1 -> Demux/1

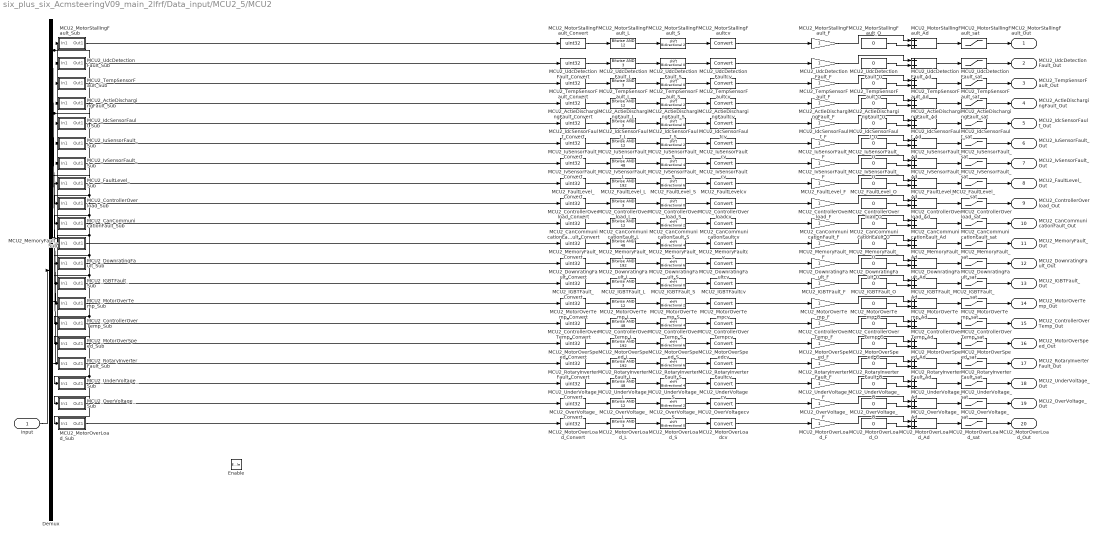
== system six_plus_six_AcmsteeringV09_main_2lfrf/Data_input/MCU2_5/MCU2 ==
  input : Inport
  Enable : EnablePort
  Demux : Demux  Outputs=8
  MCU2_ActieDischargingFault_Ad : Sum
  MCU2_ActieDischargingFault_Convert : DataTypeConversion  OutDataTypeStr=uint32
  MCU2_ActieDischargingFault_F : Gain
  MCU2_ActieDischargingFault_L : simulink/Logic and Bit Operations/Bitwise Operator  logicop=AND  UseBitMask=on  BitMask=12  BitMaskRealWorld=Stored Integer
  MCU2_ActieDischargingFault_O : Constant  Value=0  OutDataTypeStr=single
  MCU2_ActieDischargingFault_S : ArithShift  BitShiftNumber=2
  MCU2_ActieDischargingFault_Sub : Subsystem
  MCU2_ActieDischargingFault_sat : Saturate  UpperLimit=3  LowerLimit=0
  MCU2_ActieDischargingFaultcv : DataTypeConversion
  MCU2_CanCommunicationFault_Ad : Sum
  MCU2_CanCommunicationFault_Convert : DataTypeConversion  OutDataTypeStr=uint32
  MCU2_CanCommunicationFault_F : Gain
  MCU2_CanCommunicationFault_L : simulink/Logic and Bit Operations/Bitwise Operator  logicop=AND  UseBitMask=on  BitMask=12  BitMaskRealWorld=Stored Integer
  MCU2_CanCommunicationFault_O : Constant  Value=0  OutDataTypeStr=single
  MCU2_CanCommunicationFault_S : ArithShift  BitShiftNumber=2
  MCU2_CanCommunicationFault_Sub : Subsystem
  MCU2_CanCommunicationFault_sat : Saturate  UpperLimit=3  LowerLimit=0
  MCU2_CanCommunicationFaultcv : DataTypeConversion
  MCU2_ControllerOverTemp_Ad : Sum
  MCU2_ControllerOverTemp_Convert : DataTypeConversion  OutDataTypeStr=uint32
  MCU2_ControllerOverTemp_F : Gain
  MCU2_ControllerOverTemp_L : simulink/Logic and Bit Operations/Bitwise Operator  logicop=AND  UseBitMask=on  BitMask=48  BitMaskRealWorld=Stored Integer
  MCU2_ControllerOverTemp_O : Constant  Value=0  OutDataTypeStr=single
  MCU2_ControllerOverTemp_S : ArithShift  BitShiftNumber=4
  MCU2_ControllerOverTemp_Sub : Subsystem
  MCU2_ControllerOverTemp_sat : Saturate  UpperLimit=3  LowerLimit=0
  MCU2_ControllerOverTempcv : DataTypeConversion
  MCU2_ControllerOverload_Ad : Sum
  MCU2_ControllerOverload_Convert : DataTypeConversion  OutDataTypeStr=uint32
  MCU2_ControllerOverload_F : Gain
  MCU2_ControllerOverload_L : simulink/Logic and Bit Operations/Bitwise Operator  logicop=AND  UseBitMask=on  BitMask=3  BitMaskRealWorld=Stored Integer
  MCU2_ControllerOverload_O : Constant  Value=0  OutDataTypeStr=single
  MCU2_ControllerOverload_S : ArithShift
  MCU2_ControllerOverload_Sub : Subsystem
  MCU2_ControllerOverload_sat : Saturate  UpperLimit=3  LowerLimit=0
  MCU2_ControllerOverloadcv : DataTypeConversion
  MCU2_DownratingFault_Ad : Sum
  MCU2_DownratingFault_Convert : DataTypeConversion  OutDataTypeStr=uint32
  MCU2_DownratingFault_F : Gain
  MCU2_DownratingFault_L : simulink/Logic and Bit Operations/Bitwise Operator  logicop=AND  UseBitMask=on  BitMask=192  BitMaskRealWorld=Stored Integer
  MCU2_DownratingFault_O : Constant  Value=0  OutDataTypeStr=single
  MCU2_DownratingFault_S : ArithShift  BitShiftNumber=6
  MCU2_DownratingFault_Sub : Subsystem
  MCU2_DownratingFault_sat : Saturate  UpperLimit=3  LowerLimit=0
  MCU2_DownratingFaultcv : DataTypeConversion
  MCU2_FaultLevel_Ad : Sum
  MCU2_FaultLevel_Convert : DataTypeConversion  OutDataTypeStr=uint32
  MCU2_FaultLevel_F : Gain
  MCU2_FaultLevel_L : simulink/Logic and Bit Operations/Bitwise Operator  logicop=AND  UseBitMask=on  BitMask=192  BitMaskRealWorld=Stored Integer
  MCU2_FaultLevel_O : Constant  Value=0  OutDataTypeStr=single
  MCU2_FaultLevel_S : ArithShift  BitShiftNumber=6
  MCU2_FaultLevel_Sub : Subsystem
  MCU2_FaultLevel_sat : Saturate  UpperLimit=3  LowerLimit=0
  MCU2_FaultLevelcv : DataTypeConversion
  MCU2_IGBTFault_Ad : Sum
  MCU2_IGBTFault_Convert : DataTypeConversion  OutDataTypeStr=uint32
  MCU2_IGBTFault_F : Gain
  MCU2_IGBTFault_L : simulink/Logic and Bit Operations/Bitwise Operator  logicop=AND  UseBitMask=on  BitMask=3  BitMaskRealWorld=Stored Integer
  MCU2_IGBTFault_O : Constant  Value=0  OutDataTypeStr=single
  MCU2_IGBTFault_S : ArithShift
  MCU2_IGBTFault_Sub : Subsystem
  MCU2_IGBTFault_sat : Saturate  UpperLimit=3  LowerLimit=0
  MCU2_IGBTFaultcv : DataTypeConversion
  MCU2_IdcSensorFault_Ad : Sum
  MCU2_IdcSensorFault_Convert : DataTypeConversion  OutDataTypeStr=uint32
  MCU2_IdcSensorFault_F : Gain
  MCU2_IdcSensorFault_L : simulink/Logic and Bit Operations/Bitwise Operator  logicop=AND  UseBitMask=on  BitMask=3  BitMaskRealWorld=Stored Integer
  MCU2_IdcSensorFault_O : Constant  Value=0  OutDataTypeStr=single
  MCU2_IdcSensorFault_S : ArithShift
  MCU2_IdcSensorFault_Sub : Subsystem
  MCU2_IdcSensorFault_sat : Saturate  UpperLimit=3  LowerLimit=0
  MCU2_IdcSensorFaultcv : DataTypeConversion
  MCU2_IuSensorFault_Ad : Sum
  MCU2_IuSensorFault_Convert : DataTypeConversion  OutDataTypeStr=uint32
  MCU2_IuSensorFault_F : Gain
  MCU2_IuSensorFault_L : simulink/Logic and Bit Operations/Bitwise Operator  logicop=AND  UseBitMask=on  BitMask=12  BitMaskRealWorld=Stored Integer
  MCU2_IuSensorFault_O : Constant  Value=0  OutDataTypeStr=single
  MCU2_IuSensorFault_S : ArithShift  BitShiftNumber=2
  MCU2_IuSensorFault_Sub : Subsystem
  MCU2_IuSensorFault_sat : Saturate  UpperLimit=3  LowerLimit=0
  MCU2_IuSensorFaultcv : DataTypeConversion
  MCU2_IvSensorFault_Ad : Sum
  MCU2_IvSensorFault_Convert : DataTypeConversion  OutDataTypeStr=uint32
  MCU2_IvSensorFault_F : Gain
  MCU2_IvSensorFault_L : simulink/Logic and Bit Operations/Bitwise Operator  logicop=AND  UseBitMask=on  BitMask=48  BitMaskRealWorld=Stored Integer
  MCU2_IvSensorFault_O : Constant  Value=0  OutDataTypeStr=single
  MCU2_IvSensorFault_S : ArithShift  BitShiftNumber=4
  MCU2_IvSensorFault_Sub : Subsystem
  MCU2_IvSensorFault_sat : Saturate  UpperLimit=3  LowerLimit=0
  MCU2_IvSensorFaultcv : DataTypeConversion
  MCU2_MemoryFault_Ad : Sum
  MCU2_MemoryFault_Convert : DataTypeConversion  OutDataTypeStr=uint32
  MCU2_MemoryFault_F : Gain
  MCU2_MemoryFault_L : simulink/Logic and Bit Operations/Bitwise Operator  logicop=AND  UseBitMask=on  BitMask=48  BitMaskRealWorld=Stored Integer
  MCU2_MemoryFault_O : Constant  Value=0  OutDataTypeStr=single
  MCU2_MemoryFault_S : ArithShift  BitShiftNumber=4
  MCU2_MemoryFault_Sub : Subsystem
  MCU2_MemoryFault_sat : Saturate  UpperLimit=3  LowerLimit=0
  MCU2_MemoryFaultcv : DataTypeConversion
  MCU2_MotorOverLoad_Ad : Sum
  MCU2_MotorOverLoad_Convert : DataTypeConversion  OutDataTypeStr=uint32
  MCU2_MotorOverLoad_F : Gain
  MCU2_MotorOverLoad_L : simulink/Logic and Bit Operations/Bitwise Operator  logicop=AND  UseBitMask=on  BitMask=3  BitMaskRealWorld=Stored Integer
  MCU2_MotorOverLoad_O : Constant  Value=0  OutDataTypeStr=single
  MCU2_MotorOverLoad_S : ArithShift
  MCU2_MotorOverLoad_Sub : Subsystem
  MCU2_MotorOverLoad_sat : Saturate  UpperLimit=3  LowerLimit=0
  MCU2_MotorOverLoadcv : DataTypeConversion
  MCU2_MotorOverSpeed_Ad : Sum
  MCU2_MotorOverSpeed_Convert : DataTypeConversion  OutDataTypeStr=uint32
  MCU2_MotorOverSpeed_F : Gain
  MCU2_MotorOverSpeed_L : simulink/Logic and Bit Operations/Bitwise Operator  logicop=AND  UseBitMask=on  BitMask=192  BitMaskRealWorld=Stored Integer
  MCU2_MotorOverSpeed_O : Constant  Value=0  OutDataTypeStr=single
  MCU2_MotorOverSpeed_S : ArithShift  BitShiftNumber=6
  MCU2_MotorOverSpeed_Sub : Subsystem
  MCU2_MotorOverSpeed_sat : Saturate  UpperLimit=3  LowerLimit=0
  MCU2_MotorOverSpeedcv : DataTypeConversion
  MCU2_MotorOverTemp_Ad : Sum
  MCU2_MotorOverTemp_Convert : DataTypeConversion  OutDataTypeStr=uint32
  MCU2_MotorOverTemp_F : Gain
  MCU2_MotorOverTemp_L : simulink/Logic and Bit Operations/Bitwise Operator  logicop=AND  UseBitMask=on  BitMask=12  BitMaskRealWorld=Stored Integer
  MCU2_MotorOverTemp_O : Constant  Value=0  OutDataTypeStr=single
  MCU2_MotorOverTemp_S : ArithShift  BitShiftNumber=2
  MCU2_MotorOverTemp_Sub : Subsystem
  MCU2_MotorOverTemp_sat : Saturate  UpperLimit=3  LowerLimit=0
  MCU2_MotorOverTempcv : DataTypeConversion
  MCU2_MotorStallingFault_Ad : Sum
  MCU2_MotorStallingFault_Convert : DataTypeConversion  OutDataTypeStr=uint32
  MCU2_MotorStallingFault_F : Gain
  MCU2_MotorStallingFault_L : simulink/Logic and Bit Operations/Bitwise Operator  logicop=AND  UseBitMask=on  BitMask=12  BitMaskRealWorld=Stored Integer
  MCU2_MotorStallingFault_O : Constant  Value=0  OutDataTypeStr=single
  MCU2_MotorStallingFault_S : ArithShift  BitShiftNumber=2
  MCU2_MotorStallingFault_Sub : Subsystem
  MCU2_MotorStallingFault_sat : Saturate  UpperLimit=3  LowerLimit=0
  MCU2_MotorStallingFaultcv : DataTypeConversion
  MCU2_OverVoltage_Ad : Sum
  MCU2_OverVoltage_Convert : DataTypeConversion  OutDataTypeStr=uint32
  MCU2_OverVoltage_F : Gain
  MCU2_OverVoltage_L : simulink/Logic and Bit Operations/Bitwise Operator  logicop=AND  UseBitMask=on  BitMask=12  BitMaskRealWorld=Stored Integer
  MCU2_OverVoltage_O : Constant  Value=0  OutDataTypeStr=single
  MCU2_OverVoltage_S : ArithShift  BitShiftNumber=2
  MCU2_OverVoltage_Sub : Subsystem
  MCU2_OverVoltage_sat : Saturate  UpperLimit=3  LowerLimit=0
  MCU2_OverVoltagecv : DataTypeConversion
  MCU2_RotaryInverterFault_Ad : Sum
  MCU2_RotaryInverterFault_Convert : DataTypeConversion  OutDataTypeStr=uint32
  MCU2_RotaryInverterFault_F : Gain
  MCU2_RotaryInverterFault_L : simulink/Logic and Bit Operations/Bitwise Operator  logicop=AND  UseBitMask=on  BitMask=192  BitMaskRealWorld=Stored Integer
  MCU2_RotaryInverterFault_O : Constant  Value=0  OutDataTypeStr=single
  MCU2_RotaryInverterFault_S : ArithShift  BitShiftNumber=6
  MCU2_RotaryInverterFault_Sub : Subsystem
  MCU2_RotaryInverterFault_sat : Saturate  UpperLimit=3  LowerLimit=0
  MCU2_RotaryInverterFaultcv : DataTypeConversion
  MCU2_TempSensorFault_Ad : Sum
  MCU2_TempSensorFault_Convert : DataTypeConversion  OutDataTypeStr=uint32
  MCU2_TempSensorFault_F : Gain
  MCU2_TempSensorFault_L : simulink/Logic and Bit Operations/Bitwise Operator  logicop=AND  UseBitMask=on  BitMask=3  BitMaskRealWorld=Stored Integer
  MCU2_TempSensorFault_O : Constant  Value=0  OutDataTypeStr=single
  MCU2_TempSensorFault_S : ArithShift
  MCU2_TempSensorFault_Sub : Subsystem
  MCU2_TempSensorFault_sat : Saturate  UpperLimit=3  LowerLimit=0
  MCU2_TempSensorFaultcv : DataTypeConversion
  MCU2_UdcDetectionFault_Ad : Sum
  MCU2_UdcDetectionFault_Convert : DataTypeConversion  OutDataTypeStr=uint32
  MCU2_UdcDetectionFault_F : Gain
  MCU2_UdcDetectionFault_L : simulink/Logic and Bit Operations/Bitwise Operator  logicop=AND  UseBitMask=on  BitMask=3  BitMaskRealWorld=Stored Integer
  MCU2_UdcDetectionFault_O : Constant  Value=0  OutDataTypeStr=single
  MCU2_UdcDetectionFault_S : ArithShift
  MCU2_UdcDetectionFault_Sub : Subsystem
  MCU2_UdcDetectionFault_sat : Saturate  UpperLimit=3  LowerLimit=0
  MCU2_UdcDetectionFaultcv : DataTypeConversion
  MCU2_UnderVoltage_Ad : Sum
  MCU2_UnderVoltage_Convert : DataTypeConversion  OutDataTypeStr=uint32
  MCU2_UnderVoltage_F : Gain
  MCU2_UnderVoltage_L : simulink/Logic and Bit Operations/Bitwise Operator  logicop=AND  UseBitMask=on  BitMask=48  BitMaskRealWorld=Stored Integer
  MCU2_UnderVoltage_O : Constant  Value=0  OutDataTypeStr=single
  MCU2_UnderVoltage_S : ArithShift  BitShiftNumber=4
  MCU2_UnderVoltage_Sub : Subsystem
  MCU2_UnderVoltage_sat : Saturate  UpperLimit=3  LowerLimit=0
  MCU2_UnderVoltagecv : DataTypeConversion
  MCU2_MotorStallingFault_Out : Outport
  MCU2_UdcDetectionFault_Out : Outport  Port=2
  MCU2_TempSensorFault_Out : Outport  Port=3
  MCU2_ActieDischargingFault_Out : Outport  Port=4
  MCU2_IdcSensorFault_Out : Outport  Port=5
  MCU2_IuSensorFault_Out : Outport  Port=6
  MCU2_IvSensorFault_Out : Outport  Port=7
  MCU2_FaultLevel_Out : Outport  Port=8
  MCU2_ControllerOverload_Out : Outport  Port=9
  MCU2_CanCommunicationFault_Out : Outport  Port=10
  MCU2_MemoryFault_Out : Outport  Port=11
  MCU2_DownratingFault_Out : Outport  Port=12
  MCU2_IGBTFault_Out : Outport  Port=13
  MCU2_MotorOverTemp_Out : Outport  Port=14
  MCU2_ControllerOverTemp_Out : Outport  Port=15
  MCU2_MotorOverSpeed_Out : Outport  Port=16
  MCU2_RotaryInverterFault_Out : Outport  Port=17
  MCU2_UnderVoltage_Out : Outport  Port=18
  MCU2_OverVoltage_Out : Outport  Port=19
  MCU2_MotorOverLoad_Out : Outport  Port=20
  wires:
  MCU2_MotorStallingFault_F/1 -> MCU2_MotorStallingFault_Ad/1
  MCU2_MotorStallingFault_O/1 -> MCU2_MotorStallingFault_Ad/2
  MCU2_MotorStallingFault_Ad/1 -> MCU2_MotorStallingFault_sat/1
  MCU2_MotorStallingFault_sat/1 -> MCU2_MotorStallingFault_Out/1
  Demux/6 -> MCU2_MotorStallingFault_Sub/1(In1), MCU2_UdcDetectionFault_Sub/1(In1)
  MCU2_MotorStallingFault_Sub/1(Out1) -> MCU2_MotorStallingFault_Convert/1
  MCU2_MotorStallingFault_Convert/1 -> MCU2_MotorStallingFault_L/1
  MCU2_MotorStallingFault_L/1 -> MCU2_MotorStallingFault_S/1
  MCU2_MotorStallingFault_S/1 -> MCU2_MotorStallingFaultcv/1
  MCU2_MotorStallingFaultcv/1 -> MCU2_MotorStallingFault_F/1
  MCU2_UdcDetectionFault_F/1 -> MCU2_UdcDetectionFault_Ad/1
  MCU2_UdcDetectionFault_O/1 -> MCU2_UdcDetectionFault_Ad/2
  MCU2_UdcDetectionFault_Ad/1 -> MCU2_UdcDetectionFault_sat/1
  MCU2_UdcDetectionFault_sat/1 -> MCU2_UdcDetectionFault_Out/1
  MCU2_UdcDetectionFault_Sub/1(Out1) -> MCU2_UdcDetectionFault_Convert/1
  MCU2_UdcDetectionFault_Convert/1 -> MCU2_UdcDetectionFault_L/1
  MCU2_UdcDetectionFault_L/1 -> MCU2_UdcDetectionFault_S/1
  MCU2_UdcDetectionFault_S/1 -> MCU2_UdcDetectionFaultcv/1
  MCU2_UdcDetectionFaultcv/1 -> MCU2_UdcDetectionFault_F/1
  MCU2_TempSensorFault_F/1 -> MCU2_TempSensorFault_Ad/1
  MCU2_TempSensorFault_O/1 -> MCU2_TempSensorFault_Ad/2
  MCU2_TempSensorFault_Ad/1 -> MCU2_TempSensorFault_sat/1
  MCU2_TempSensorFault_sat/1 -> MCU2_TempSensorFault_Out/1
  Demux/5 -> MCU2_TempSensorFault_Sub/1(In1), MCU2_ActieDischargingFault_Sub/1(In1)
  MCU2_TempSensorFault_Sub/1(Out1) -> MCU2_TempSensorFault_Convert/1
  MCU2_TempSensorFault_Convert/1 -> MCU2_TempSensorFault_L/1
  MCU2_TempSensorFault_L/1 -> MCU2_TempSensorFault_S/1
  MCU2_TempSensorFault_S/1 -> MCU2_TempSensorFaultcv/1
  MCU2_TempSensorFaultcv/1 -> MCU2_TempSensorFault_F/1
  MCU2_ActieDischargingFault_F/1 -> MCU2_ActieDischargingFault_Ad/1
  MCU2_ActieDischargingFault_O/1 -> MCU2_ActieDischargingFault_Ad/2
  MCU2_ActieDischargingFault_Ad/1 -> MCU2_ActieDischargingFault_sat/1
  MCU2_ActieDischargingFault_sat/1 -> MCU2_ActieDischargingFault_Out/1
  MCU2_ActieDischargingFault_Sub/1(Out1) -> MCU2_ActieDischargingFault_Convert/1
  MCU2_ActieDischargingFault_Convert/1 -> MCU2_ActieDischargingFault_L/1
  MCU2_ActieDischargingFault_L/1 -> MCU2_ActieDischargingFault_S/1
  MCU2_ActieDischargingFault_S/1 -> MCU2_ActieDischargingFaultcv/1
  MCU2_ActieDischargingFaultcv/1 -> MCU2_ActieDischargingFault_F/1
  MCU2_IdcSensorFault_F/1 -> MCU2_IdcSensorFault_Ad/1
  MCU2_IdcSensorFault_O/1 -> MCU2_IdcSensorFault_Ad/2
  MCU2_IdcSensorFault_Ad/1 -> MCU2_IdcSensorFault_sat/1
  MCU2_IdcSensorFault_sat/1 -> MCU2_IdcSensorFault_Out/1
  Demux/4 -> MCU2_IdcSensorFault_Sub/1(In1), MCU2_IuSensorFault_Sub/1(In1), MCU2_IvSensorFault_Sub/1(In1), MCU2_FaultLevel_Sub/1(In1)
  MCU2_IdcSensorFault_Sub/1(Out1) -> MCU2_IdcSensorFault_Convert/1
  MCU2_IdcSensorFault_Convert/1 -> MCU2_IdcSensorFault_L/1
  MCU2_IdcSensorFault_L/1 -> MCU2_IdcSensorFault_S/1
  MCU2_IdcSensorFault_S/1 -> MCU2_IdcSensorFaultcv/1
  MCU2_IdcSensorFaultcv/1 -> MCU2_IdcSensorFault_F/1
  MCU2_IuSensorFault_F/1 -> MCU2_IuSensorFault_Ad/1
  MCU2_IuSensorFault_O/1 -> MCU2_IuSensorFault_Ad/2
  MCU2_IuSensorFault_Ad/1 -> MCU2_IuSensorFault_sat/1
  MCU2_IuSensorFault_sat/1 -> MCU2_IuSensorFault_Out/1
  MCU2_IuSensorFault_Sub/1(Out1) -> MCU2_IuSensorFault_Convert/1
  MCU2_IuSensorFault_Convert/1 -> MCU2_IuSensorFault_L/1
  MCU2_IuSensorFault_L/1 -> MCU2_IuSensorFault_S/1
  MCU2_IuSensorFault_S/1 -> MCU2_IuSensorFaultcv/1
  MCU2_IuSensorFaultcv/1 -> MCU2_IuSensorFault_F/1
  MCU2_IvSensorFault_F/1 -> MCU2_IvSensorFault_Ad/1
  MCU2_IvSensorFault_O/1 -> MCU2_IvSensorFault_Ad/2
  MCU2_IvSensorFault_Ad/1 -> MCU2_IvSensorFault_sat/1
  MCU2_IvSensorFault_sat/1 -> MCU2_IvSensorFault_Out/1
  MCU2_IvSensorFault_Sub/1(Out1) -> MCU2_IvSensorFault_Convert/1
  MCU2_IvSensorFault_Convert/1 -> MCU2_IvSensorFault_L/1
  MCU2_IvSensorFault_L/1 -> MCU2_IvSensorFault_S/1
  MCU2_IvSensorFault_S/1 -> MCU2_IvSensorFaultcv/1
  MCU2_IvSensorFaultcv/1 -> MCU2_IvSensorFault_F/1
  MCU2_FaultLevel_F/1 -> MCU2_FaultLevel_Ad/1
  MCU2_FaultLevel_O/1 -> MCU2_FaultLevel_Ad/2
  MCU2_FaultLevel_Ad/1 -> MCU2_FaultLevel_sat/1
  MCU2_FaultLevel_sat/1 -> MCU2_FaultLevel_Out/1
  MCU2_FaultLevel_Sub/1(Out1) -> MCU2_FaultLevel_Convert/1
  MCU2_FaultLevel_Convert/1 -> MCU2_FaultLevel_L/1
  MCU2_FaultLevel_L/1 -> MCU2_FaultLevel_S/1
  MCU2_FaultLevel_S/1 -> MCU2_FaultLevelcv/1
  MCU2_FaultLevelcv/1 -> MCU2_FaultLevel_F/1
  MCU2_ControllerOverload_F/1 -> MCU2_ControllerOverload_Ad/1
  MCU2_ControllerOverload_O/1 -> MCU2_ControllerOverload_Ad/2
  MCU2_ControllerOverload_Ad/1 -> MCU2_ControllerOverload_sat/1
  MCU2_ControllerOverload_sat/1 -> MCU2_ControllerOverload_Out/1
  Demux/1 -> MCU2_UnderVoltage_Sub/1(In1), MCU2_OverVoltage_Sub/1(In1), MCU2_ControllerOverload_Sub/1(In1), MCU2_RotaryInverterFault_Sub/1(In1)
  MCU2_ControllerOverload_Sub/1(Out1) -> MCU2_ControllerOverload_Convert/1
  MCU2_ControllerOverload_Convert/1 -> MCU2_ControllerOverload_L/1
  MCU2_ControllerOverload_L/1 -> MCU2_ControllerOverload_S/1
  MCU2_ControllerOverload_S/1 -> MCU2_ControllerOverloadcv/1
  MCU2_ControllerOverloadcv/1 -> MCU2_ControllerOverload_F/1
  MCU2_CanCommunicationFault_F/1 -> MCU2_CanCommunicationFault_Ad/1
  MCU2_CanCommunicationFault_O/1 -> MCU2_CanCommunicationFault_Ad/2
  MCU2_CanCommunicationFault_Ad/1 -> MCU2_CanCommunicationFault_sat/1
  MCU2_CanCommunicationFault_sat/1 -> MCU2_CanCommunicationFault_Out/1
  Demux/3 -> MCU2_DownratingFault_Sub/1(In1), MCU2_MotorOverLoad_Sub/1(In1), MCU2_MemoryFault_Sub/1(In1), MCU2_CanCommunicationFault_Sub/1(In1)
  MCU2_CanCommunicationFault_Sub/1(Out1) -> MCU2_CanCommunicationFault_Convert/1
  MCU2_CanCommunicationFault_Convert/1 -> MCU2_CanCommunicationFault_L/1
  MCU2_CanCommunicationFault_L/1 -> MCU2_CanCommunicationFault_S/1
  MCU2_CanCommunicationFault_S/1 -> MCU2_CanCommunicationFaultcv/1
  MCU2_CanCommunicationFaultcv/1 -> MCU2_CanCommunicationFault_F/1
  MCU2_MemoryFault_F/1 -> MCU2_MemoryFault_Ad/1
  MCU2_MemoryFault_O/1 -> MCU2_MemoryFault_Ad/2
  MCU2_MemoryFault_Ad/1 -> MCU2_MemoryFault_sat/1
  MCU2_MemoryFault_sat/1 -> MCU2_MemoryFault_Out/1
  MCU2_MemoryFault_Sub/1(Out1) -> MCU2_MemoryFault_Convert/1
  MCU2_MemoryFault_Convert/1 -> MCU2_MemoryFault_L/1
  MCU2_MemoryFault_L/1 -> MCU2_MemoryFault_S/1
  MCU2_MemoryFault_S/1 -> MCU2_MemoryFaultcv/1
  MCU2_MemoryFaultcv/1 -> MCU2_MemoryFault_F/1
  MCU2_DownratingFault_F/1 -> MCU2_DownratingFault_Ad/1
  MCU2_DownratingFault_O/1 -> MCU2_DownratingFault_Ad/2
  MCU2_DownratingFault_Ad/1 -> MCU2_DownratingFault_sat/1
  MCU2_DownratingFault_sat/1 -> MCU2_DownratingFault_Out/1
  MCU2_DownratingFault_Sub/1(Out1) -> MCU2_DownratingFault_Convert/1
  MCU2_DownratingFault_Convert/1 -> MCU2_DownratingFault_L/1
  MCU2_DownratingFault_L/1 -> MCU2_DownratingFault_S/1
  MCU2_DownratingFault_S/1 -> MCU2_DownratingFaultcv/1
  MCU2_DownratingFaultcv/1 -> MCU2_DownratingFault_F/1
  MCU2_IGBTFault_F/1 -> MCU2_IGBTFault_Ad/1
  MCU2_IGBTFault_O/1 -> MCU2_IGBTFault_Ad/2
  MCU2_IGBTFault_Ad/1 -> MCU2_IGBTFault_sat/1
  MCU2_IGBTFault_sat/1 -> MCU2_IGBTFault_Out/1
  Demux/2 -> MCU2_ControllerOverTemp_Sub/1(In1), MCU2_MotorOverSpeed_Sub/1(In1), MCU2_IGBTFault_Sub/1(In1), MCU2_MotorOverTemp_Sub/1(In1)
  MCU2_IGBTFault_Sub/1(Out1) -> MCU2_IGBTFault_Convert/1
  MCU2_IGBTFault_Convert/1 -> MCU2_IGBTFault_L/1
  MCU2_IGBTFault_L/1 -> MCU2_IGBTFault_S/1
  MCU2_IGBTFault_S/1 -> MCU2_IGBTFaultcv/1
  MCU2_IGBTFaultcv/1 -> MCU2_IGBTFault_F/1
  MCU2_MotorOverTemp_F/1 -> MCU2_MotorOverTemp_Ad/1
  MCU2_MotorOverTemp_O/1 -> MCU2_MotorOverTemp_Ad/2
  MCU2_MotorOverTemp_Ad/1 -> MCU2_MotorOverTemp_sat/1
  MCU2_MotorOverTemp_sat/1 -> MCU2_MotorOverTemp_Out/1
  MCU2_MotorOverTemp_Sub/1(Out1) -> MCU2_MotorOverTemp_Convert/1
  MCU2_MotorOverTemp_Convert/1 -> MCU2_MotorOverTemp_L/1
  MCU2_MotorOverTemp_L/1 -> MCU2_MotorOverTemp_S/1
  MCU2_MotorOverTemp_S/1 -> MCU2_MotorOverTempcv/1
  MCU2_MotorOverTempcv/1 -> MCU2_MotorOverTemp_F/1
  MCU2_ControllerOverTemp_F/1 -> MCU2_ControllerOverTemp_Ad/1
  MCU2_ControllerOverTemp_O/1 -> MCU2_ControllerOverTemp_Ad/2
  MCU2_ControllerOverTemp_Ad/1 -> MCU2_ControllerOverTemp_sat/1
  MCU2_ControllerOverTemp_sat/1 -> MCU2_ControllerOverTemp_Out/1
  MCU2_ControllerOverTemp_Sub/1(Out1) -> MCU2_ControllerOverTemp_Convert/1
  MCU2_ControllerOverTemp_Convert/1 -> MCU2_ControllerOverTemp_L/1
  MCU2_ControllerOverTemp_L/1 -> MCU2_ControllerOverTemp_S/1
  MCU2_ControllerOverTemp_S/1 -> MCU2_ControllerOverTempcv/1
  MCU2_ControllerOverTempcv/1 -> MCU2_ControllerOverTemp_F/1
  MCU2_MotorOverSpeed_F/1 -> MCU2_MotorOverSpeed_Ad/1
  MCU2_MotorOverSpeed_O/1 -> MCU2_MotorOverSpeed_Ad/2
  MCU2_MotorOverSpeed_Ad/1 -> MCU2_MotorOverSpeed_sat/1
  MCU2_MotorOverSpeed_sat/1 -> MCU2_MotorOverSpeed_Out/1
  MCU2_MotorOverSpeed_Sub/1(Out1) -> MCU2_MotorOverSpeed_Convert/1
  MCU2_MotorOverSpeed_Convert/1 -> MCU2_MotorOverSpeed_L/1
  MCU2_MotorOverSpeed_L/1 -> MCU2_MotorOverSpeed_S/1
  MCU2_MotorOverSpeed_S/1 -> MCU2_MotorOverSpeedcv/1
  MCU2_MotorOverSpeedcv/1 -> MCU2_MotorOverSpeed_F/1
  MCU2_RotaryInverterFault_F/1 -> MCU2_RotaryInverterFault_Ad/1
  MCU2_RotaryInverterFault_O/1 -> MCU2_RotaryInverterFault_Ad/2
  MCU2_RotaryInverterFault_Ad/1 -> MCU2_RotaryInverterFault_sat/1
  MCU2_RotaryInverterFault_sat/1 -> MCU2_RotaryInverterFault_Out/1
  MCU2_RotaryInverterFault_Sub/1(Out1) -> MCU2_RotaryInverterFault_Convert/1
  MCU2_RotaryInverterFault_Convert/1 -> MCU2_RotaryInverterFault_L/1
  MCU2_RotaryInverterFault_L/1 -> MCU2_RotaryInverterFault_S/1
  MCU2_RotaryInverterFault_S/1 -> MCU2_RotaryInverterFaultcv/1
  MCU2_RotaryInverterFaultcv/1 -> MCU2_RotaryInverterFault_F/1
  MCU2_UnderVoltage_F/1 -> MCU2_UnderVoltage_Ad/1
  MCU2_UnderVoltage_O/1 -> MCU2_UnderVoltage_Ad/2
  MCU2_UnderVoltage_Ad/1 -> MCU2_UnderVoltage_sat/1
  MCU2_UnderVoltage_sat/1 -> MCU2_UnderVoltage_Out/1
  MCU2_UnderVoltage_Sub/1(Out1) -> MCU2_UnderVoltage_Convert/1
  MCU2_UnderVoltage_Convert/1 -> MCU2_UnderVoltage_L/1
  MCU2_UnderVoltage_L/1 -> MCU2_UnderVoltage_S/1
  MCU2_UnderVoltage_S/1 -> MCU2_UnderVoltagecv/1
  MCU2_UnderVoltagecv/1 -> MCU2_UnderVoltage_F/1
  MCU2_OverVoltage_F/1 -> MCU2_OverVoltage_Ad/1
  MCU2_OverVoltage_O/1 -> MCU2_OverVoltage_Ad/2
  MCU2_OverVoltage_Ad/1 -> MCU2_OverVoltage_sat/1
  MCU2_OverVoltage_sat/1 -> MCU2_OverVoltage_Out/1
  MCU2_OverVoltage_Sub/1(Out1) -> MCU2_OverVoltage_Convert/1
  MCU2_OverVoltage_Convert/1 -> MCU2_OverVoltage_L/1
  MCU2_OverVoltage_L/1 -> MCU2_OverVoltage_S/1
  MCU2_OverVoltage_S/1 -> MCU2_OverVoltagecv/1
  MCU2_OverVoltagecv/1 -> MCU2_OverVoltage_F/1
  MCU2_MotorOverLoad_F/1 -> MCU2_MotorOverLoad_Ad/1
  MCU2_MotorOverLoad_O/1 -> MCU2_MotorOverLoad_Ad/2
  MCU2_MotorOverLoad_Ad/1 -> MCU2_MotorOverLoad_sat/1
  MCU2_MotorOverLoad_sat/1 -> MCU2_MotorOverLoad_Out/1
  MCU2_MotorOverLoad_Sub/1(Out1) -> MCU2_MotorOverLoad_Convert/1
  MCU2_MotorOverLoad_Convert/1 -> MCU2_MotorOverLoad_L/1
  MCU2_MotorOverLoad_L/1 -> MCU2_MotorOverLoad_S/1
  MCU2_MotorOverLoad_S/1 -> MCU2_MotorOverLoadcv/1
  MCU2_MotorOverLoadcv/1 -> MCU2_MotorOverLoad_F/1
  input/1 -> Demux/1

== matlab function six_plus_six_AcmsteeringV09_main_2lfrf/Data_input/1/Enabled
Subsystem/MATLAB Function1 ==
  data: current_in input; current_out output
function current_out = motec_current(current_in)
    if current_in>32768
        current_out=current_in-65535;
    else
        current_out=current_in;
    end
end

== matlab function six_plus_six_AcmsteeringV09_main_2lfrf/MainControl/mode_control/forward/forward/Drive/驱动防滑控制TCS/直行TCS/直行/MATLAB Function1 ==
  data: s_act_lr input; flag_lr output; s_opt_zhuan input; s_opt_zhuan_add input; flag_lr_pre input int8
function flag_lr = fcn(s_act_lr,s_opt_zhuan,s_opt_zhuan_add,flag_lr_pre)
%#codegen
if s_act_lr>s_opt_zhuan+s_opt_zhuan_add
    flag_lr=int8(1);
elseif s_act_lr<s_opt_zhuan
    flag_lr =int8(0);
else
    flag_lr=int8(flag_lr_pre);
end
end
